simulink model "FM_Mod_Self_Module_Sawtooth"  (R2018b)
settings: Solver=VariableStepAuto  StartTime=0.0  StopTime=2*10^-3  MaxStep=0.0001  MinStep=0.001  RelTol=1e-3
undefined symbols (not defined in the file or in its folder): DiscIntNeverNeededParam
settings Model: Creator=lenovo  LastModifiedBy=lenovo
settings DataIOCC: ExternalInput=tt, t  TimeSaveName=tmax

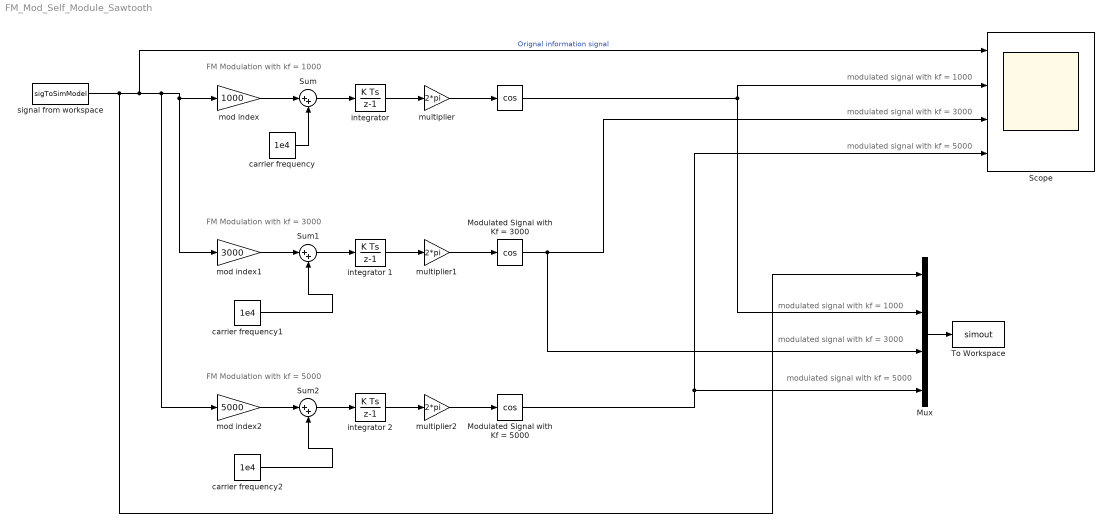
== system FM_Mod_Self_Module_Sawtooth ==
  note: FM Modulation with kf = 1000
  note: modulated signal with kf = 1000
  note: FM Modulation with kf = 3000
  note: FM Modulation with kf = 5000
  note: modulated signal with kf = 3000
  note: modulated signal with kf = 5000
  note: modulated signal with kf = 1000
  note: modulated signal with kf = 3000
  note: modulated signal with kf = 5000
  " " : Trigonometry  Operator=cos
  Modulated Signal with Kf = 3000 : Trigonometry  Operator=cos
  Modulated Signal with Kf = 5000 : Trigonometry  Operator=cos
  Mux : Mux
  Scope : Scope  NumInputPorts=4
  Sum : Sum  Inputs=|++
  Sum1 : Sum  Inputs=|++
  Sum2 : Sum  Inputs=|++
  To Workspace : ToWorkspace  VariableName=simout  SaveFormat=Timeseries  SampleTime=-1
  carrier frequency : Constant  Value=1e4
  carrier frequency1 : Constant  Value=1e4
  carrier frequency2 : Constant  Value=1e4
  "integrator " : DiscreteIntegrator  SampleTime=1/1000000  ICPrevOutput=DiscIntNeverNeededParam  ICPrevScaledInput=DiscIntNeverNeededParam
  integrator 1 : DiscreteIntegrator  SampleTime=1/1000000  ICPrevOutput=DiscIntNeverNeededParam  ICPrevScaledInput=DiscIntNeverNeededParam
  integrator 2 : DiscreteIntegrator  SampleTime=1/1000000  ICPrevOutput=DiscIntNeverNeededParam  ICPrevScaledInput=DiscIntNeverNeededParam
  mod index : Gain  Gain=1000
  mod index1 : Gain  Gain=3000
  mod index2 : Gain  Gain=5000
  multiplier : Gain  Gain=2*pi
  multiplier1 : Gain  Gain=2*pi
  multiplier2 : Gain  Gain=2*pi
  signal from workspace : FromWorkspace  VariableName=sigToSimModel  SampleTime=0
  wires:
  signal from workspace/1 -> Mux/1, Scope/1, mod index2/1, mod index1/1, mod index/1  "Orignal information signal"
  Mux/1 -> To Workspace/1
  carrier frequency1/1 -> Sum1/2
  integrator 1/1 -> multiplier1/1
  multiplier1/1 -> Modulated Signal with Kf = 3000/1
  mod index1/1 -> Sum1/1
  Sum1/1 -> integrator 1/1
  Sum2/1 -> integrator 2/1
  mod index2/1 -> Sum2/1
  multiplier2/1 -> Modulated Signal with Kf = 5000/1
  integrator 2/1 -> multiplier2/1
  carrier frequency2/1 -> Sum2/2
  Modulated Signal with Kf = 3000/1 -> Mux/3, Scope/3
  Modulated Signal with Kf = 5000/1 -> Mux/4, Scope/4
  " "/1 -> Mux/2, Scope/2
  carrier frequency/1 -> Sum/2
  "integrator "/1 -> multiplier/1
  mod index/1 -> Sum/1
  Sum/1 -> "integrator "/1
  multiplier/1 -> " "/1
